simulink model "LAVM_openloop"  (R2022b)
settings: Solver=FixedStepDiscrete  StartTime=0.0  StopTime=0.1  FixedStep=Tsim  MaxStep=Tsim  RelTol=1e-7
values from neighbouring files (symbols this model uses):
  flux = 0.025    [LAVM_openloop.sldd]
  J = 4.982E-8    [LAVM_openloop.sldd]
  ka = 0.027    [LAVM_openloop.sldd]
  kc = 0.008    [LAVM_openloop.sldd]
  L_com = 0.00094    [LAVM_openloop.sldd]
  L_dif = 6.0E-5    [LAVM_openloop.sldd]
  R = 4.27    [LAVM_openloop.sldd]
  Tpwm = 0.0001    [LAVM_openloop.sldd]
  Tsim = 1.0E-6    [LAVM_openloop.sldd]
  Udc = 3.7    [LAVM_openloop.sldd]
undefined symbols (not defined in the file or in its folder): DiscIntNeverNeededParam
libraries: spsDCVoltageSourceLib x1, spsControlledCurrentSourceLib x1, spsVoltageMeasurementLib x1, simulink x1, spsUniversalBridgeLib x1, spspowerguiLib x1
settings Model: DataDictionary=LAVM_openloop.sldd  Creator=SSC  LastModifiedBy=SSC

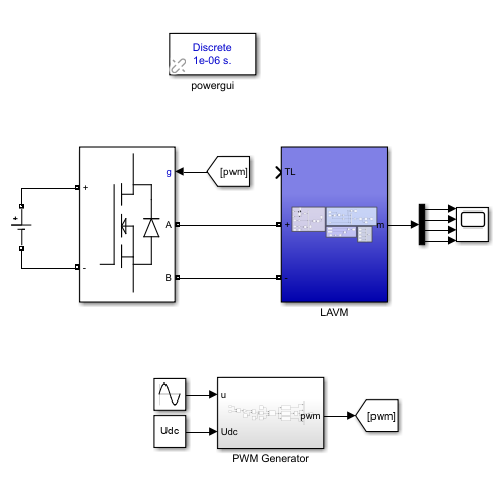
[thumbnail: Simulink's stored preview of the top-level diagram]
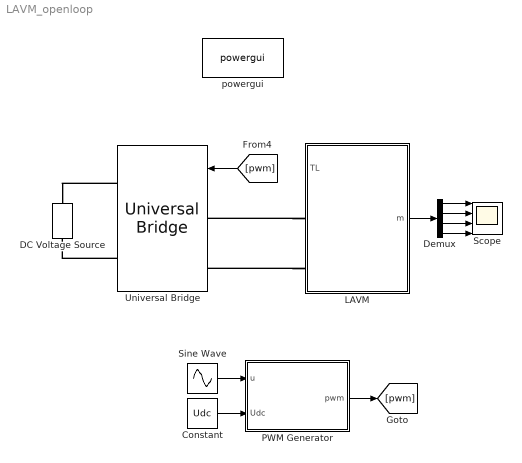
== system LAVM_openloop ==
  Constant : Constant  Value=Udc
  DC Voltage Source : spsDCVoltageSourceLib/DC Voltage Source  Amplitude=Udc  Measurements=None
  Demux : Demux
  LAVM : Subsystem
  PWM Generator : Subsystem
  Scope : Scope  NumInputPorts=4
  Sine Wave : Sin  Amplitude=2.5  Frequency=183*2*pi
  Universal Bridge : spsUniversalBridgeLib/Universal Bridge  Arms=2  SnubberResistance=1e5  SnubberCapacitance=inf  Device=MOSFET / Diodes  Ron=1e-3  Lon=0  ForwardVoltages="[  0  0  ]"  ForwardVoltage=0  GTOparameters=[ 10e-6 , 20e-6 ]  IGBTparameters=[ 1e-6 , 2e-6 ]  Measurements=None  Measurements_2=None  converterType=Rectifier
  powergui : spspowerguiLib/powergui  Priority=1  SimulationMode=Discrete  SampleTime=Tsim  frequency=60  Iterations=50  frequencyindice=0  Pbase=100e6  ErrMax=1e-4  UnitsV=kV  UnitsW=MW  buscounter=0  FunctionMessages=off  echomessages=off  EnableUseOfTLC=off  CurrentSourceSwitches=off  DisableSnubberDevices=off  DisableRonSwitches=off  DisableVfSwitches=off  DisplayEquations=off  AutomaticDiscreteSolvers=off  SolverType=Tustin/Backward Euler (TBE)  Interpol=off  ExternalGateDelay=off  methode=off  Ts=100  x0status=blocks  SPID=on  SwTol=0  HookPort=off  NonlinearTolerance=1e-4  nMaxIteration=100  ContinueOnMaxIteration=off  RestoreLinks=warning  ResistiveCurrentMeasurement=off  Frange=[0:2:500]  Ylog=off  Xlog=on  ShowGrid=off  save=off  variable=ZData  structure=0  ZoomFFT=off  StartTime=0.0  cycles=1  DisplayStyle=1  fundamental=60  FreqAxis=off  MaxFrequency=1000  frequencyindicesteady=1  RmsSteady=1  display=off
  wires:
  LAVM/1(m) -> Demux/1
  Demux/1 -> Scope/1
  Demux/2 -> Scope/2
  Demux/3 -> Scope/3
  Demux/4 -> Scope/4
  [pwm] -> Universal Bridge/1
  PWM Generator/1(pwm) -> [pwm]
  Sine Wave/1 -> PWM Generator/1(u)
  Constant/1 -> PWM Generator/2(Udc)
  connections:
  Universal Bridge/RConn1 -- DC Voltage Source/RConn1
  Universal Bridge/RConn2 -- DC Voltage Source/LConn1
  LAVM/LConn1 -- Universal Bridge/LConn1
  LAVM/LConn2 -- Universal Bridge/LConn2

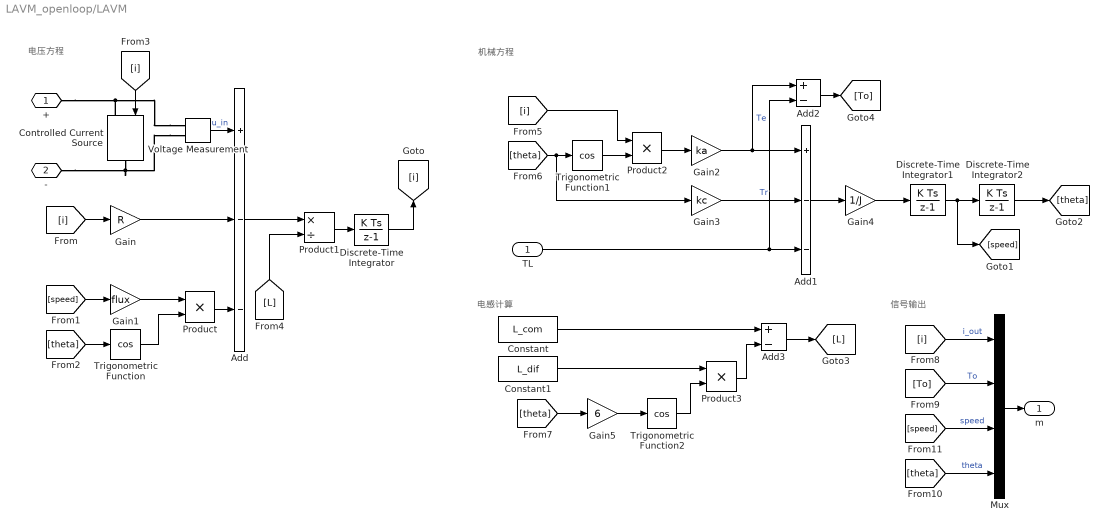
== system LAVM_openloop/LAVM ==
  note: 信号输出
  note: 电感计算
  note: 机械方程
  note: 电压方程
  TL : Inport
  Add : Sum  Inputs=+--
  Add1 : Sum  Inputs=+--
  Add2 : Sum  Inputs=+-
  Add3 : Sum  Inputs=+-
  Constant : Constant  Value=L_com
  Constant1 : Constant  Value=L_dif
  Controlled Current Source : spsControlledCurrentSourceLib/Controlled Current Source  Initialize=on  Source_Type=AC  Amplitude=0  Phase=0  Frequency=0  Measurements=None
  Discrete-Time Integrator : DiscreteIntegrator  SampleTime=-1  ICPrevOutput=DiscIntNeverNeededParam  ICPrevScaledInput=DiscIntNeverNeededParam
  Discrete-Time Integrator1 : DiscreteIntegrator  SampleTime=-1  ICPrevOutput=DiscIntNeverNeededParam  ICPrevScaledInput=DiscIntNeverNeededParam
  Discrete-Time Integrator2 : DiscreteIntegrator  SampleTime=-1  ICPrevOutput=DiscIntNeverNeededParam  ICPrevScaledInput=DiscIntNeverNeededParam
  Gain : Gain  Gain=R
  Gain1 : Gain  Gain=flux
  Gain2 : Gain  Gain=ka
  Gain3 : Gain  Gain=kc
  Gain4 : Gain  Gain=1/J
  Gain5 : Gain  Gain=6
  Mux : Mux
  Product : Product
  Product1 : Product  Inputs=*/
  Product2 : Product
  Product3 : Product
  Trigonometric Function : Trigonometry  Operator=cos
  Trigonometric Function1 : Trigonometry  Operator=cos
  Trigonometric Function2 : Trigonometry  Operator=cos
  Voltage Measurement : spsVoltageMeasurementLib/Voltage Measurement  PhasorSimulation=off  OutputType=Complex  PSBequivalent=0
  + : PMIOPort  Side=Left
  - : PMIOPort  Port=2  Side=Left
  m : Outport
  wires:
  Product1/1 -> Discrete-Time Integrator/1
  [speed] -> Gain1/1
  [i] -> Controlled Current Source/1
  [L] -> Product1/2
  Add/1 -> Product1/1
  Discrete-Time Integrator/1 -> [i]
  [i] -> Gain/1
  Product/1 -> Add/3
  Gain/1 -> Add/2
  Trigonometric Function/1 -> Product/2
  Gain1/1 -> Product/1
  [theta] -> Trigonometric Function/1
  Voltage Measurement/1 -> Add/1  "u_in"
  [theta] -> Gain3/1, Trigonometric Function1/1
  [i] -> Product2/1
  Trigonometric Function1/1 -> Product2/2
  Product2/1 -> Gain2/1
  Gain2/1 -> Add2/1, Add1/1  "Te"
  Gain3/1 -> Add1/2  "Tr"
  TL/1 -> Add2/2, Add1/3
  Add1/1 -> Gain4/1
  Gain4/1 -> Discrete-Time Integrator1/1
  Discrete-Time Integrator1/1 -> [speed], Discrete-Time Integrator2/1
  Discrete-Time Integrator2/1 -> [theta]
  Constant/1 -> Add3/1
  [theta] -> Gain5/1
  Gain5/1 -> Trigonometric Function2/1
  Trigonometric Function2/1 -> Product3/2
  Constant1/1 -> Product3/1
  Product3/1 -> Add3/2
  Add3/1 -> [L]
  [i] -> Mux/1  "i_out"
  Add2/1 -> [To]
  [theta] -> Mux/4  "theta"
  [speed] -> Mux/3  "speed"
  [To] -> Mux/2  "To"
  Mux/1 -> m/1
  connections:
  Voltage Measurement/LConn1 -- +/RConn1 -- Controlled Current Source/LConn1
  Voltage Measurement/LConn2 -- -/RConn1 -- Controlled Current Source/RConn1

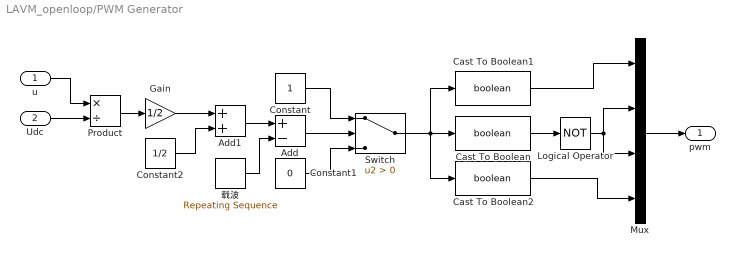
== system LAVM_openloop/PWM Generator ==
  u : Inport
  Udc : Inport  Port=2
  Add : Sum  Inputs=+-
  Add1 : Sum
  Cast To Boolean : DataTypeConversion  OutDataTypeStr=boolean  SaturateOnIntegerOverflow=off  RndMeth=Floor
  Cast To Boolean1 : DataTypeConversion  OutDataTypeStr=boolean  SaturateOnIntegerOverflow=off  RndMeth=Floor
  Cast To Boolean2 : DataTypeConversion  OutDataTypeStr=boolean  SaturateOnIntegerOverflow=off  RndMeth=Floor
  Constant : Constant
  Constant1 : Constant  Value=0
  Constant2 : Constant  Value=1/2
  Gain : Gain  Gain=1/2
  Logical Operator : Logic  Operator=NOT  AllPortsSameDT=off  OutDataTypeStr=boolean
  Mux : Mux
  Product : Product  Inputs=*/
  Switch : Switch  Criteria=u2 > Threshold  SaturateOnIntegerOverflow=off  InputSameDT=off
  载波 : simulink/Sources/Repeating Sequence  rep_seq_t=[0 0.5*Tpwm Tpwm]  rep_seq_y=[0 1 0]
  pwm : Outport
  wires:
  Switch/1 -> Cast To Boolean2/1, Cast To Boolean/1, Cast To Boolean1/1
  Cast To Boolean2/1 -> Mux/4
  Mux/1 -> pwm/1
  Logical Operator/1 -> Mux/2, Mux/3
  Constant/1 -> Switch/1
  载波/1 -> Add/2
  Cast To Boolean1/1 -> Mux/1
  Constant1/1 -> Switch/3
  Cast To Boolean/1 -> Logical Operator/1
  u/1 -> Product/1
  Udc/1 -> Product/2
  Product/1 -> Gain/1
  Gain/1 -> Add1/1
  Constant2/1 -> Add1/2
  Add1/1 -> Add/1
  Add/1 -> Switch/2
